simulink model "tank_prop_controller"  (R2013a)
settings: Solver=ode45  StartTime=0.0  StopTime=100  RelTol=1e-3
undefined symbols (not defined in the file): A, ka, ke, kv, n, R
settings Model: Creator=Ahmed  LastModifiedBy=Ahmed

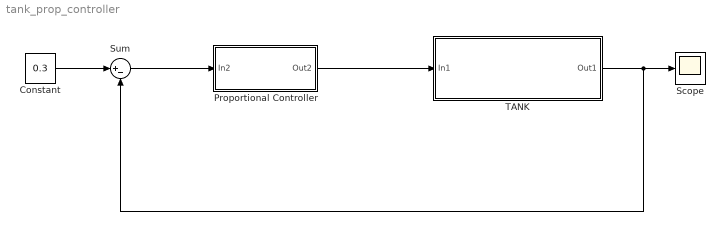
== system tank_prop_controller ==
  Constant : Constant  Value=0.3
  Proportional Controller : Subsystem
  Scope : Scope
  Sum : Sum  Inputs=|+-
  TANK : Subsystem
  wires:
  TANK/1(Out1) -> Sum/2, Scope/1
  Constant/1 -> Sum/1
  Sum/1 -> Proportional Controller/1(In2)
  Proportional Controller/1(Out2) -> TANK/1(In1)

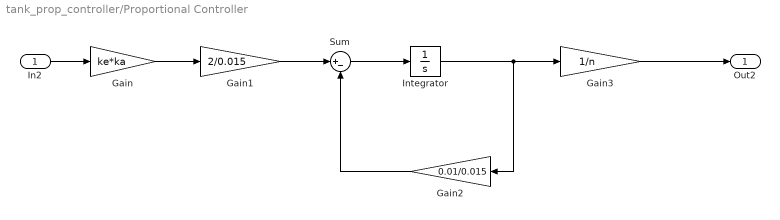
== system tank_prop_controller/Proportional Controller ==
  In2 : Inport
  Gain : Gain  Gain=ke*ka
  Gain1 : Gain  Gain=2/0.015
  Gain2 : Gain  Gain=0.01/0.015
  Gain3 : Gain  Gain=1/n
  Integrator : Integrator
  Sum : Sum  Inputs=|+-
  Out2 : Outport
  wires:
  In2/1 -> Gain/1
  Gain/1 -> Gain1/1
  Gain1/1 -> Sum/1
  Sum/1 -> Integrator/1
  Integrator/1 -> Gain3/1, Gain2/1
  Gain2/1 -> Sum/2
  Gain3/1 -> Out2/1

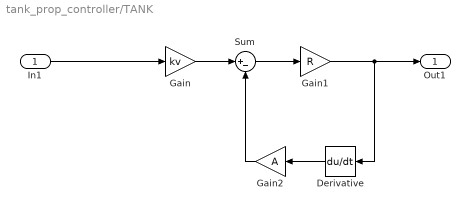
== system tank_prop_controller/TANK ==
  In1 : Inport
  Derivative : Derivative
  Gain : Gain  Gain=kv
  Gain1 : Gain  Gain=R
  Gain2 : Gain  Gain=A
  Sum : Sum  Inputs=|+-
  Out1 : Outport
  wires:
  Derivative/1 -> Gain2/1
  Gain/1 -> Sum/1
  Gain1/1 -> Out1/1, Derivative/1
  In1/1 -> Gain/1
  Sum/1 -> Gain1/1
  Gain2/1 -> Sum/2
